simulink model "Phase_shift_Test"  (R2022b)
settings: Solver=VariableStepAuto  StartTime=0.0  StopTime=5  MaxStep=1e-4  RelTol=1e-3
settings Model: Creator=admin  LastModifiedBy=admin

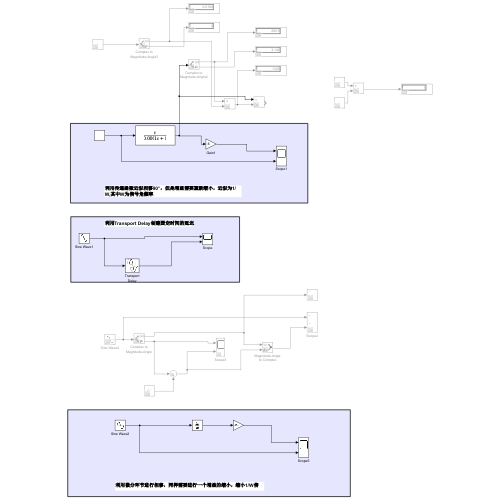
[thumbnail: Simulink's stored preview of the top-level diagram]
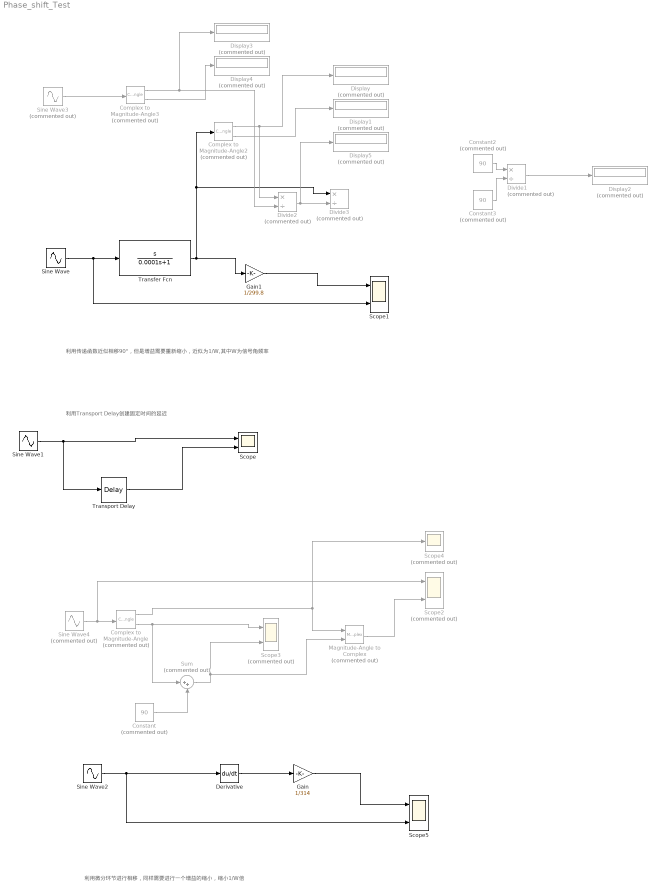
== system Phase_shift_Test ==
  note: 利用微分环节进行相移，同样需要进行一个增益的缩小，缩小1/W倍
  note: 利用传递函数近似相移90°，但是增益需要重新缩小，近似为1/W,其中W为信号角频率
  note: 利用Transport Delay创建固定时间的延迟
  Complex to Magnitude-Angle : ComplexToMagnitudeAngle  Commented=on
  Complex to Magnitude-Angle2 : ComplexToMagnitudeAngle  Commented=on
  Complex to Magnitude-Angle3 : ComplexToMagnitudeAngle  Commented=on
  Constant : Constant  Commented=on  Value=90
  Constant2 : Constant  Commented=on  Value=90
  Constant3 : Constant  Commented=on  Value=90
  Derivative : Derivative
  Display{,1..5} (6 alike) : Display  Commented=on
  Divide1 : Product  Commented=on  Inputs=*/
  Divide2 : Product  Commented=on  Inputs=*/
  Divide3 : Product  Commented=on  Inputs=*/
  Gain : Gain  Gain=1/314
  Gain1 : Gain  Gain=1/299.8
  Magnitude-Angle to Complex : MagnitudeAngleToComplex  Commented=on
  Scope : Scope  NumInputPorts=2
  Scope1 : Scope  NumInputPorts=2
  Scope2 : Scope  Commented=on  NumInputPorts=2
  Scope3 : Scope  Commented=on  NumInputPorts=2
  Scope4 : Scope  Commented=on
  Scope5 : Scope  NumInputPorts=2
  Sine Wave : Sin  Frequency=300  SampleTime=0
  Sine Wave1 : Sin  Frequency=2*pi*50  Samples=100  SampleTime=0
  Sine Wave2 : Sin  Frequency=2*pi*50  Samples=100  SampleTime=0
  Sine Wave3 : Sin  Commented=on  Frequency=300  SampleTime=0
  Sine Wave4 : Sin  Commented=on  Frequency=2*pi*50  Samples=100  SampleTime=0
  Sum : Sum  Commented=on  Inputs=|++
  Transfer Fcn : TransferFcn  Numerator=[1 0]  Denominator=[0.0001 1]
  Transport Delay : TransportDelay  DelayTime=0.005
  wires:
  Sine Wave/1 -> Scope1/2, Transfer Fcn/1
  Sine Wave1/1 -> Transport Delay/1, Scope/1
  Transport Delay/1 -> Scope/2
  Sine Wave2/1 -> Scope5/2, Derivative/1
  Sum/1 -> Scope3/2, Magnitude-Angle to Complex/2
  Complex to Magnitude-Angle/2 -> Scope3/1, Sum/1
  Complex to Magnitude-Angle/1 -> Scope4/1, Magnitude-Angle to Complex/1
  Magnitude-Angle to Complex/1 -> Scope2/2
  Constant/1 -> Sum/2
  Derivative/1 -> Gain/1
  Gain/1 -> Scope5/1
  Transfer Fcn/1 -> Divide3/1, Complex to Magnitude-Angle2/1, Gain1/1
  Constant2/1 -> Divide1/1
  Constant3/1 -> Divide1/2
  Divide1/1 -> Display2/1
  Complex to Magnitude-Angle2/1 -> Divide2/1, Display/1
  Complex to Magnitude-Angle2/2 -> Display1/1
  Sine Wave3/1 -> Complex to Magnitude-Angle3/1
  Complex to Magnitude-Angle3/1 -> Divide2/2, Display3/1
  Complex to Magnitude-Angle3/2 -> Display4/1
  Divide2/1 -> Divide3/2, Display5/1
  Gain1/1 -> Scope1/1
  Sine Wave4/1 -> Scope2/1, Complex to Magnitude-Angle/1
